simulink model "mrac_model_quad_linear"  (R2021b)
settings: Solver=VariableStepAuto  StartTime=0.0  StopTime=5  RelTol=1e-3
values from neighbouring files (symbols this model uses):
  A = reshape([mt1,mt2,mt3,mt4,mt5,mt6,mt7,mt8],12,12)    [Jacob.m]    (also in Lineared_SS_model.m = reshape([-1.097500e-06;0.000000e+00;0.000000e+00;-4.432200e-; find_optimal_lqr.m = reshape([-1.097500e-06;0.000000e+00;0.000000e+00;-4.432200e-; start_drone.m = zeros(12))
  B = reshape([mt9,mt10],12,4)    [Jacob.m]    (also in Lineared_SS_model.m = reshape([0.000000e+00;0.000000e+00;0.000000e+00;0.000000e+00; find_optimal_lqr.m = reshape([0.000000e+00;0.000000e+00;0.000000e+00;0.000000e+00; nlStateFcn.m = [0 0 0]; start_drone.m = zeros(12,4))
libraries: slctrlblks x1
settings Model: Creator=Elena  LastModifiedBy=Elena

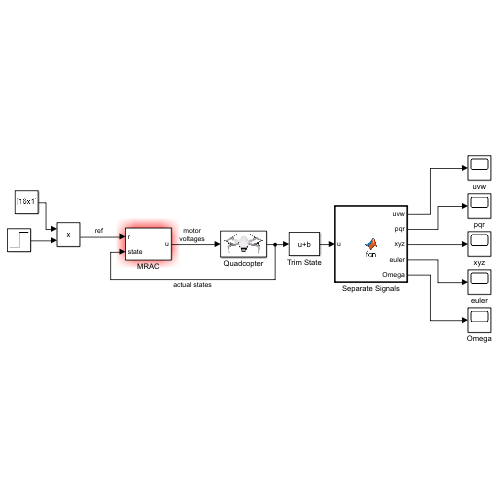
[thumbnail: Simulink's stored preview of the top-level diagram]
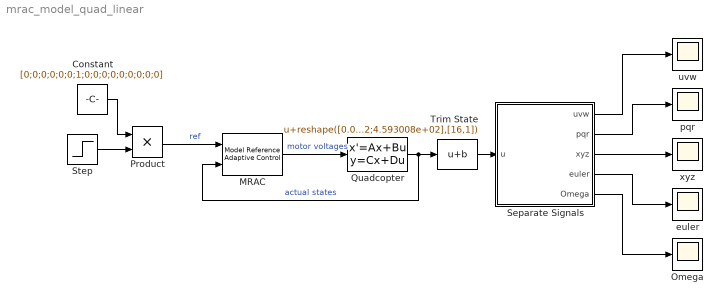
== system mrac_model_quad_linear ==
  Constant : Constant  Value=[0;0;0;0;0;0;1;0;0;0;0;0;0;0;0;0]
  MRAC : slctrlblks/Model Reference Adaptive Control  A=A  B=B  Am=Am  Bm=Bm  kx=0  FBLrEnable=on  gamma_kx=1  FBLrEnableMod=on  kr=0  FFLrEnable=on  gamma_kr=1  FFLrEnableMod=on  AdaptEnable=on  gamma=1  WLrEnableMod=on  Q=1  FeatureTypeOptions=State  nCen=20  cSpanMin=-1  cSpanMax=1  cSig=5  adaptiveCntrlOutport=off  modChoice=None  sigma_val=0.1
      settings: SourceProductBaseCode=SD
  Omega : Scope
  Product : Product
  Quadcopter : StateSpace  A=A  B=B  C=eye(16)  D=zeros(16,4)  InitialCondition=0
      mask Display: image('drone_model.png'); % Use "Edit Image" on toolstrip to change.
  Separate Signals : MATLAB Function  TreatAsAtomicUnit=on
  Step : Step  SampleTime=0
  Trim State : Bias  Bias=reshape([0.000000e+00;0.000000e+00;0.000000e+00;0.000000e+00;0.000000e+00;0.000000e+00;0.000000e+00;0.000000e+00;0.000000e+00;0.000000e+00;0.000000e+00;0.000000e+00;4.593008e+02;4.593008e+02;4.593008e+02;4.593008e+02],[16,1])
  euler : Scope
  pqr : Scope
  uvw : Scope
  xyz : Scope
  wires:
  Step/1 -> Product/2
  Quadcopter/1 -> MRAC/2, Trim State/1  "actual states"
  Constant/1 -> Product/1
  Product/1 -> MRAC/1  "ref"
  Separate Signals/3(xyz) -> xyz/1
  Separate Signals/2(pqr) -> pqr/1
  Separate Signals/1(uvw) -> uvw/1
  Separate Signals/4(euler) -> euler/1
  Separate Signals/5(Omega) -> Omega/1
  MRAC/1 -> Quadcopter/1  "motor voltages"
  Trim State/1 -> Separate Signals/1(u)

== matlab function mrac_model_quad_linear/Separate Signals ==
  data: u input; uvw output; pqr output; xyz output; euler output; Omega output
function [uvw,pqr,xyz,euler,Omega] = fcn(u)

uvw=u(1:3);
pqr=u((1:3)+3);
xyz=u((1:3)+6);
euler=u((1:3)+9);
Omega=u((1:4)+12);
